simulink model "ComunicacionMATLABhomeIO_P4"  (R2023b)
settings: Solver=VariableStepAuto  StartTime=0.0  StopTime=450000  RelTol=1e-3
libraries: realtime_pacer_lib x1
settings Model: Creator=usuario  LastModifiedBy=juanl_00e1ytj
settings SolverCC: AlgebraicLoopSolver=TrustRegion
settings DebuggingCC: UnconnectedInputMsg=warning  UnconnectedOutputMsg=warning  UnconnectedLineMsg=warning
settings ModelReferenceCC: EnableRefExpFcnMdlSchedulingChecks=on
settings RTWCC: DLArmComputeVersion=19.05

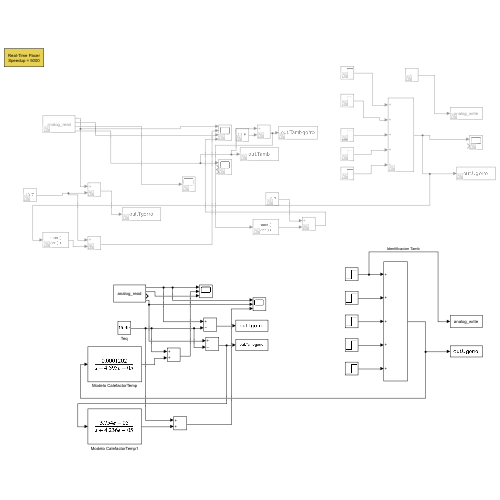
[thumbnail: Simulink's stored preview of the top-level diagram]
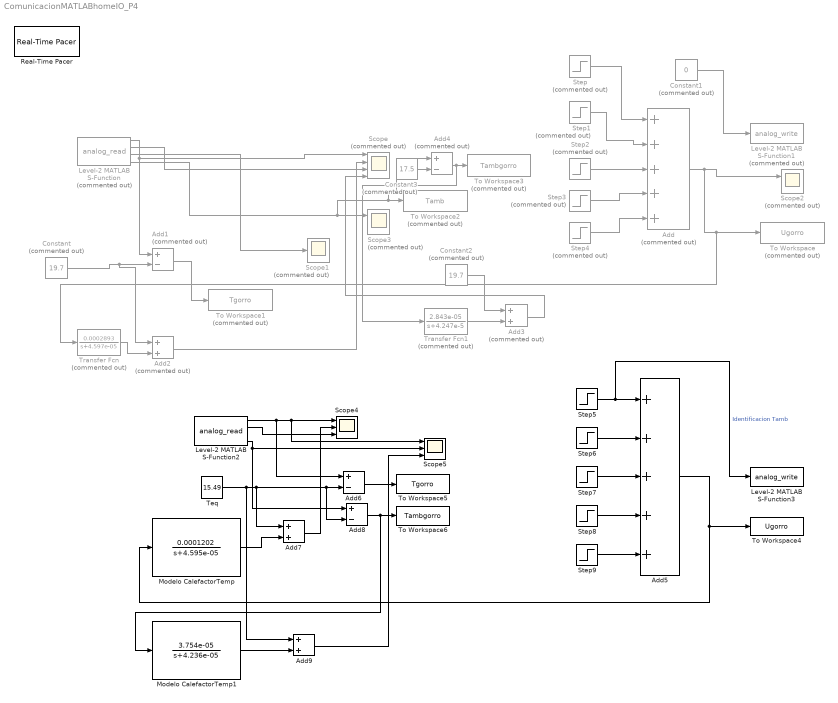
== system ComunicacionMATLABhomeIO_P4 ==
  Add : Sum  Commented=on  Inputs=+++++
  Add1 : Sum  Commented=on  Inputs=+-
  Add2 : Sum  Commented=on
  Add3 : Sum  Commented=on
  Add4 : Sum  Commented=on  Inputs=+-
  Add5 : Sum  Inputs=+++++
  Add6 : Sum  Inputs=+-
  Add7 : Sum
  Add8 : Sum  Inputs=+-
  Add9 : Sum
  Constant : Constant  Commented=on  Value=19.7
  Constant1 : Constant  Commented=on  Value=0
  Constant2 : Constant  Commented=on  Value=19.7
  Constant3 : Constant  Commented=on  Value=17.5
  Level-2 MATLAB S-Function : M-S-Function  Commented=on  FunctionName=analog_read
  Level-2 MATLAB S-Function1 : M-S-Function  Commented=on  FunctionName=analog_write
  Level-2 MATLAB S-Function2 : M-S-Function  FunctionName=analog_read
  Level-2 MATLAB S-Function3 : M-S-Function  FunctionName=analog_write
  Modelo CalefactorTemp : TransferFcn  Numerator=[0.0001202]  Denominator=[1 4.595e-05]
  Modelo CalefactorTemp1 : TransferFcn  Numerator=[3.754e-05]  Denominator=[1 4.236e-05]
  Real-Time Pacer : realtime_pacer_lib/Real-Time Pacer  simTimePerRealTime=5000
      settings: SourceProductName=Real-Time Pacer
  Scope : Scope  Commented=on  NumInputPorts=4
  Scope1 : Scope  Commented=on
  Scope2 : Scope  Commented=on  NumInputPorts=2
  Scope3 : Scope  Commented=on  NumInputPorts=3
  Scope4 : Scope  NumInputPorts=3
  Scope5 : Scope  NumInputPorts=3
  Step : Step  Commented=on  Time=0  After=0  SampleTime=0
  Step1 : Step  Commented=on  Time=20000  SampleTime=0
  Step2 : Step  Commented=on  Time=85000  After=2  SampleTime=0
  Step3 : Step  Commented=on  Time=190000  After=3  SampleTime=0
  Step4 : Step  Commented=on  Time=300000  After=3  SampleTime=0
  Step5 : Step  Time=0  After=0  SampleTime=0
  Step6 : Step  Time=20000  SampleTime=0
  Step7 : Step  Time=85000  After=2  SampleTime=0
  Step8 : Step  Time=190000  After=3  SampleTime=0
  Step9 : Step  Time=300000  After=3  SampleTime=0
  Teq : Constant  Value=15.49
  To Workspace : ToWorkspace  Commented=on  VariableName=Ugorro  SampleTime=-1
  To Workspace1 : ToWorkspace  Commented=on  VariableName=Tgorro  SampleTime=-1
  To Workspace2 : ToWorkspace  Commented=on  VariableName=Tamb  SampleTime=-1
  To Workspace3 : ToWorkspace  Commented=on  VariableName=Tambgorro  SampleTime=-1
  To Workspace4 : ToWorkspace  VariableName=Ugorro  SampleTime=-1
  To Workspace5 : ToWorkspace  VariableName=Tgorro  SampleTime=-1
  To Workspace6 : ToWorkspace  VariableName=Tambgorro  SampleTime=-1
  Transfer Fcn : TransferFcn  Commented=on  Numerator=[0.0002893]  Denominator=[1 4.597e-05]
  Transfer Fcn1 : TransferFcn  Commented=on  Numerator=[2.843e-05]  Denominator=[1 4.247e-5]
  wires:
  Level-2 MATLAB S-Function/1 -> Scope/1, Add1/1
  Step/1 -> Add/1
  Add/1 -> Transfer Fcn/1, To Workspace/1, Scope2/1
  Step1/1 -> Add/2
  Level-2 MATLAB S-Function/3 -> Scope1/1
  Level-2 MATLAB S-Function/2 -> Scope/3
  Step4/1 -> Add/5
  Step3/1 -> Add/4
  Step2/1 -> Add/3
  Constant/1 -> Add2/1, Add1/2
  Add1/1 -> To Workspace1/1
  Transfer Fcn/1 -> Add2/2
  Add2/1 -> Scope/2
  Level-2 MATLAB S-Function/4 -> Add4/1, To Workspace2/1, Scope3/1
  Constant1/1 -> Level-2 MATLAB S-Function1/1
  Constant2/1 -> Add3/1
  Transfer Fcn1/1 -> Add3/2
  Add3/1 -> Scope/4
  Add4/1 -> Transfer Fcn1/1, To Workspace3/1
  Constant3/1 -> Add4/2
  Level-2 MATLAB S-Function2/1 -> Scope5/1, Scope4/1, Add6/1
  Level-2 MATLAB S-Function2/2 -> Scope4/3
  Step5/1 -> Level-2 MATLAB S-Function3/1, Add5/1  "Identificacion Tamb"
  Step6/1 -> Add5/2
  Step7/1 -> Add5/3
  Step9/1 -> Add5/5
  Step8/1 -> Add5/4
  Add5/1 -> Modelo CalefactorTemp/1, To Workspace4/1
  Teq/1 -> Add9/1, Add7/1, Add8/2, Add6/2
  Add6/1 -> To Workspace5/1
  Modelo CalefactorTemp/1 -> Add7/2
  Add7/1 -> Scope4/2
  Add8/1 -> Modelo CalefactorTemp1/1, To Workspace6/1
  Level-2 MATLAB S-Function2/4 -> Add8/1, Scope5/2
  Modelo CalefactorTemp1/1 -> Add9/2
  Add9/1 -> Scope5/3
